simulink model "completo"  (R2022b)
settings: Solver=ode5  StartTime=0.0  StopTime=20  FixedStep=0.0001  RelTol=1e-3
InitFcn:
  | params_completo
values from neighbouring files (symbols this model uses):
  a = 1/tau    (= 1000)    [params_completo.m]
  A = [0, -a ... (first row only)    [params_completo.m]
  A_h = 0.4297    [params_completo.m]
  alpha = 40    [params_completo.m]
  b = dp/tau    (= 10000)    [params_completo.m]
  C = [1, 0]    [params_completo.m]
  k1 = 700    [params_completo.m]
  k2 = 500    [params_completo.m]
  kap1 = 1800    [params_completo.m]
  kappa = 200    [params_completo.m]
  Q = [6000 0 ... (first row only)    [params_completo.m]
  theta = 2000    [params_completo.m]
undefined symbols (not defined in the file or in its folder): B_h, cp, freq, G_h
settings Model: Creator=gerar  LastModifiedBy=Gerardo
settings SolverCC: AlgebraicLoopSolver=TrustRegion
settings DebuggingCC: UnconnectedInputMsg=warning  UnconnectedOutputMsg=warning  UnconnectedLineMsg=warning  SFMachineParentedDataDiag=warning
settings ModelReferenceCC: EnableRefExpFcnMdlSchedulingChecks=on
settings SFSimCC: CustomCodeUndefinedFunction=UseInterfaceOnly

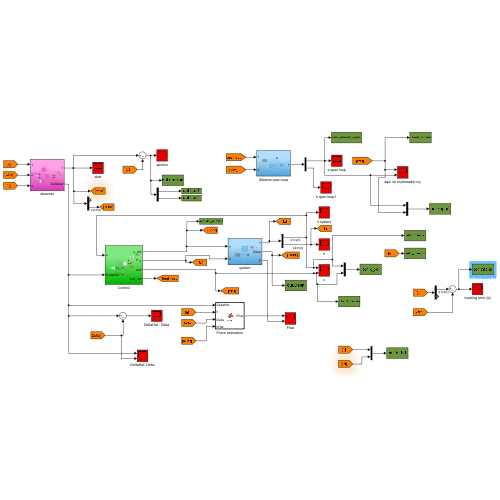
[thumbnail: Simulink's stored preview of the top-level diagram]
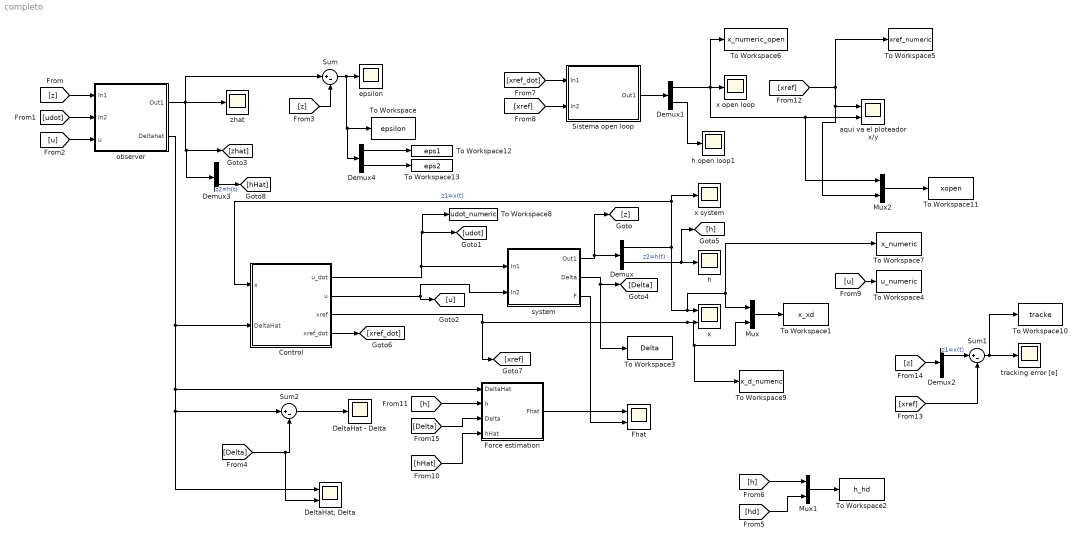
== system completo ==
  Control : Subsystem
  DeltaHat - Delta : Scope
  "DeltaHat, Delta" : Scope  NumInputPorts=2
  Demux{,1..4} (5 alike) : Demux  Outputs=2
  Fhat : Scope  NumInputPorts=2
  Force estimation : MATLAB Function  TreatAsAtomicUnit=on
  Mux : Mux  Inputs=2
  Mux1 : Mux  Inputs=2
  Mux2 : Mux  Inputs=2
  Sistema open loop : Subsystem
  Sum : Sum  Inputs=|+-
  Sum1 : Sum  Inputs=|+-
  Sum2 : Sum  Inputs=|+-
  To Workspace : ToWorkspace  VariableName=epsilon  SaveFormat=Timeseries  SampleTime=-1
  To Workspace1 : ToWorkspace  VariableName=x_xd  SaveFormat=Timeseries  SampleTime=-1
  To Workspace10 : ToWorkspace  VariableName=tracke  SaveFormat=Timeseries  SampleTime=-1
  To Workspace11 : ToWorkspace  VariableName=xopen  SaveFormat=Timeseries  SampleTime=-1
  To Workspace12 : ToWorkspace  VariableName=eps1  SaveFormat=Timeseries  SampleTime=-1
  To Workspace13 : ToWorkspace  VariableName=eps2  SaveFormat=Timeseries  SampleTime=-1
  To Workspace2 : ToWorkspace  VariableName=h_hd  SaveFormat=Timeseries  SampleTime=-1
  To Workspace3 : ToWorkspace  VariableName=Delta  SaveFormat=Timeseries  SampleTime=-1
  To Workspace4 : ToWorkspace  VariableName=u_numeric  SaveFormat=Structure  SampleTime=-1
  To Workspace5 : ToWorkspace  VariableName=xref_numeric  SaveFormat=Structure  SampleTime=-1
  To Workspace6 : ToWorkspace  VariableName=x_numeric_open  SaveFormat=Structure  SampleTime=-1
  To Workspace7 : ToWorkspace  VariableName=x_numeric  SaveFormat=Structure  SampleTime=-1
  To Workspace8 : ToWorkspace  VariableName=udot_numeric  SaveFormat=Structure  SampleTime=-1
  To Workspace9 : ToWorkspace  VariableName=x_d_numeric  SaveFormat=Structure  SampleTime=-1
  aqui va el ploteador x/y : Scope  NumInputPorts=2
  epsilon : Scope
  h : Scope
  h open loop1 : Scope
  observer : Subsystem
  system : Subsystem
  tracking error [e] : Scope
  x : Scope  NumInputPorts=2
  x open loop : Scope
  x system : Scope
  zhat : Scope
  wires:
  Control/1(u_dot) -> To Workspace8/1, [udot], system/1(In1)
  Control/2(u) -> system/2(In2), [u]
  Control/3(xref) -> [xref], To Workspace9/1, Mux/2, x/2
  Demux/2 -> [h], h/1  "z2=h(t)"
  Demux/1 -> Mux/1, To Workspace7/1, x/1, x system/1, Control/1(x)  "z1=x(t)"
  system/1(Out1) -> Demux/1, [z]
  [z] -> observer/1(In1)
  observer/1(Out1) -> Demux3/1, [zhat], zhat/1, Sum/1
  [udot] -> observer/2(In2)
  [u] -> observer/3(u)
  [z] -> Sum/2
  Sum/1 -> Demux4/1, To Workspace/1, epsilon/1
  Mux/1 -> To Workspace1/1
  [h] -> Mux1/1
  [hd] -> Mux1/2
  Mux1/1 -> To Workspace2/1
  Control/4(xref_dot) -> [xref_dot]
  [xref_dot] -> Sistema open loop/1(In1)
  [xref] -> Sistema open loop/2(In2)
  Sistema open loop/1(Out1) -> Demux1/1
  Demux1/2 -> h open loop1/1
  Demux1/1 -> To Workspace6/1, x open loop/1, Mux2/1, aqui va el ploteador x/y/2
  [u] -> To Workspace4/1
  [xref] -> To Workspace5/1, Mux2/2, aqui va el ploteador x/y/1
  Mux2/1 -> To Workspace11/1
  [z] -> Demux2/1
  Demux2/1 -> Sum1/1  "z1=x(t)"
  [xref] -> Sum1/2
  Sum1/1 -> To Workspace10/1, tracking error [e]/1
  observer/2(Deltahat) -> "DeltaHat, Delta"/1, Sum2/1, Force estimation/1(DeltaHat), Control/2(DeltaHat)
  system/2(Delta) -> To Workspace3/1, [Delta]
  [Delta] -> "DeltaHat, Delta"/2, Sum2/2
  Sum2/1 -> DeltaHat - Delta/1
  Force estimation/1(Fhat) -> Fhat/1
  Demux3/2 -> [hHat]  "z2=h(t)"
  [hHat] -> Force estimation/4(hHat)
  system/3(F) -> Fhat/2
  [h] -> Force estimation/2(h)
  [Delta] -> Force estimation/3(Delta)
  Demux4/1 -> To Workspace12/1
  Demux4/2 -> To Workspace13/1

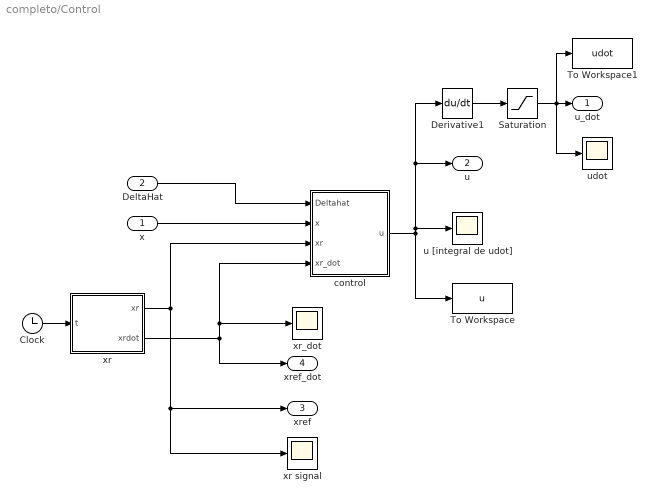
== system completo/Control ==
  x : Inport
  DeltaHat : Inport  Port=2
  Clock : Clock
  Derivative1 : Derivative
  Saturation : Saturate  UpperLimit=100  LowerLimit=-100
  To Workspace : ToWorkspace  VariableName=u  SaveFormat=Timeseries  SampleTime=-1
  To Workspace1 : ToWorkspace  VariableName=udot  SaveFormat=Timeseries  SampleTime=-1
  control : MATLAB Function  TreatAsAtomicUnit=on
  u [integral de udot] : Scope
  udot : Scope
  xr : MATLAB Function  TreatAsAtomicUnit=on
  xr signal : Scope
  xr_dot : Scope
  u_dot : Outport  VectorParamsAs1DForOutWhenUnconnected=off
  u : Outport  Port=2  VectorParamsAs1DForOutWhenUnconnected=off
  xref : Outport  Port=3  VectorParamsAs1DForOutWhenUnconnected=off
  xref_dot : Outport  Port=4  VectorParamsAs1DForOutWhenUnconnected=off
  wires:
  x/1 -> control/2(x)
  Clock/1 -> xr/1(t)
  xr/1(xr) -> xr signal/1, xref/1, control/3(xr)
  xr/2(xrdot) -> xref_dot/1, xr_dot/1, control/4(xr_dot)
  control/1(u) -> Derivative1/1, u/1, u [integral de udot]/1, To Workspace/1
  Derivative1/1 -> Saturation/1
  Saturation/1 -> To Workspace1/1, udot/1, u_dot/1
  DeltaHat/1 -> control/1(Deltahat)

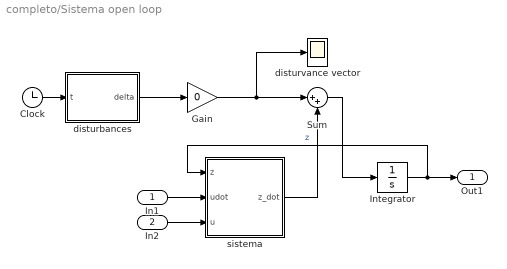
== system completo/Sistema open loop ==
  In1 : Inport
  In2 : Inport  Port=2
  Clock : Clock
  Gain : Gain  Gain=0
  Integrator : Integrator  InitialCondition=[3;-2]
  Sum : Sum  Inputs=|++
  disturbances : MATLAB Function  TreatAsAtomicUnit=on
  disturvance vector : Scope
  sistema : MATLAB Function  TreatAsAtomicUnit=on
  Out1 : Outport  VectorParamsAs1DForOutWhenUnconnected=off
  wires:
  Integrator/1 -> Out1/1, sistema/1(z)  "z"
  In1/1 -> sistema/2(udot)
  In2/1 -> sistema/3(u)
  Clock/1 -> disturbances/1(t)
  sistema/1(z_dot) -> Sum/2
  disturbances/1(delta) -> Gain/1
  Sum/1 -> Integrator/1
  Gain/1 -> Sum/1, disturvance vector/1

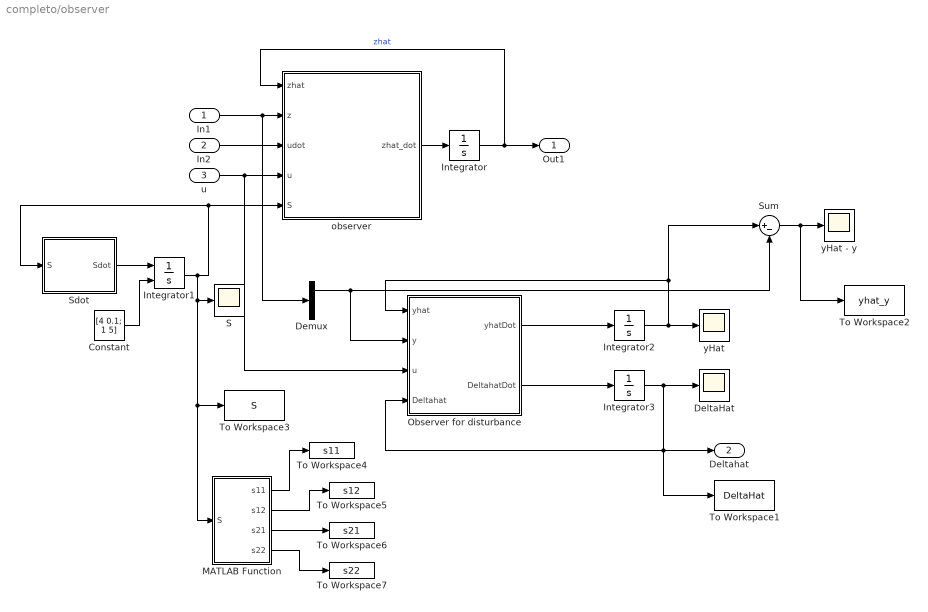
== system completo/observer ==
  In1 : Inport
  In2 : Inport  Port=2
  u : Inport  Port=3
  Constant : Constant  Value=[4 0.1; 1 5]
  DeltaHat : Scope
  Demux : Demux  Outputs=2
  Integrator : Integrator  InitialCondition=[0;0]
  Integrator1 : Integrator  InitialConditionSource=external
  Integrator2 : Integrator
  Integrator3 : Integrator
  MATLAB Function : MATLAB Function  TreatAsAtomicUnit=on
  Observer for disturbance : MATLAB Function  TreatAsAtomicUnit=on
  S : Scope
  Sdot : MATLAB Function  TreatAsAtomicUnit=on
  Sum : Sum  Inputs=|+-
  To Workspace1 : ToWorkspace  VariableName=DeltaHat  SaveFormat=Timeseries  SampleTime=-1
  To Workspace2 : ToWorkspace  VariableName=yhat_y  SaveFormat=Timeseries  SampleTime=-1
  To Workspace3 : ToWorkspace  VariableName=S  SaveFormat=Timeseries  SampleTime=-1
  To Workspace4 : ToWorkspace  VariableName=s11  SaveFormat=Timeseries  SampleTime=-1
  To Workspace5 : ToWorkspace  VariableName=s12  SaveFormat=Timeseries  SampleTime=-1
  To Workspace6 : ToWorkspace  VariableName=s21  SaveFormat=Timeseries  SampleTime=-1
  To Workspace7 : ToWorkspace  VariableName=s22  SaveFormat=Timeseries  SampleTime=-1
  observer : MATLAB Function  TreatAsAtomicUnit=on
  yHat : Scope
  yHat - y : Scope
  Out1 : Outport  VectorParamsAs1DForOutWhenUnconnected=off
  Deltahat : Outport  Port=2  VectorParamsAs1DForOutWhenUnconnected=off
  wires:
  observer/1(zhat_dot) -> Integrator/1
  Integrator/1 -> observer/1(zhat), Out1/1  "zhat"
  In1/1 -> Demux/1, observer/2(z)
  In2/1 -> observer/3(udot)
  u/1 -> Observer for disturbance/3(u), observer/4(u)
  Constant/1 -> Integrator1/2
  Sdot/1(Sdot) -> Integrator1/1
  Integrator1/1 -> MATLAB Function/1(S), To Workspace3/1, S/1, Sdot/1(S), observer/5(S)
  Observer for disturbance/1(yhatDot) -> Integrator2/1
  Observer for disturbance/2(DeltahatDot) -> Integrator3/1
  Integrator2/1 -> yHat/1, Sum/1, Observer for disturbance/1(yhat)
  Integrator3/1 -> DeltaHat/1, To Workspace1/1, Observer for disturbance/4(Deltahat), Deltahat/1
  Demux/1 -> Sum/2, Observer for disturbance/2(y)
  Sum/1 -> To Workspace2/1, yHat - y/1
  MATLAB Function/1(s11) -> To Workspace4/1
  MATLAB Function/2(s12) -> To Workspace5/1
  MATLAB Function/3(s21) -> To Workspace6/1
  MATLAB Function/4(s22) -> To Workspace7/1

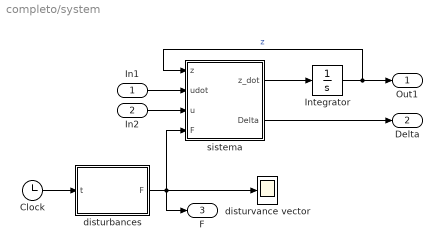
== system completo/system ==
  In1 : Inport
  In2 : Inport  Port=2
  Clock : Clock
  Integrator : Integrator  InitialCondition=[3;-2]
  disturbances : MATLAB Function  TreatAsAtomicUnit=on
  disturvance vector : Scope
  sistema : MATLAB Function  TreatAsAtomicUnit=on
  Out1 : Outport  VectorParamsAs1DForOutWhenUnconnected=off
  Delta : Outport  Port=2  VectorParamsAs1DForOutWhenUnconnected=off
  F : Outport  Port=3  VectorParamsAs1DForOutWhenUnconnected=off
  wires:
  Integrator/1 -> Out1/1, sistema/1(z)  "z"
  In1/1 -> sistema/2(udot)
  In2/1 -> sistema/3(u)
  Clock/1 -> disturbances/1(t)
  disturbances/1(F) -> F/1, sistema/4(F), disturvance vector/1
  sistema/1(z_dot) -> Integrator/1
  sistema/2(Delta) -> Delta/1

== matlab function completo/Sistema open loop/disturbances ==
  data: t input; delta output
function delta = dist(t)

delta_x = 30;
delta_h = 25*sin(t); %2*sin(t); -- causa error en el observer

delta = [delta_x ; delta_h];

== matlab function completo/Sistema open loop/sistema ==
  data: z input; udot input; u input; z_dot output; A parameter; A_h parameter; B_h parameter; G_h parameter; a parameter; b parameter
function z_dot = sys(z, udot, u, A, A_h, B_h, G_h, a, b)

gx = [ - a*z(1,1) + b*u ; 
       A_h*udot - B_h*abs(udot)*z(2,1) - G_h*udot*abs(z(2,1))];

z_dot = A*z + gx ;

== matlab function completo/observer/Sdot ==
  data: S input; Sdot output; a parameter; C parameter; theta parameter; Q parameter
function Sdot = fcn(S, a, C, theta, Q)

A_ = [ 0 -a ; 
       0  0 ];

Sdot = - theta*S - A_'*S - S*A_ + Q*(C'*C);

== matlab function completo/observer/Observer for disturbance ==
  data: yhat input; y input; u input; Deltahat input; yhatDot output; DeltahatDot output; b parameter; k1 parameter; k2 parameter; a parameter
function [yhatDot, DeltahatDot] = fcn(yhat, y, u, Deltahat, b, k1, k2, a)

yhatDot = - a*yhat + b*u + Deltahat - k1*(yhat - y);
DeltahatDot = - (yhat - y) + (k2)*(k2 - a - k1)*(yhat - y) ;

== matlab function completo/observer/MATLAB Function ==
  data: S input; s11 output; s12 output; s21 output; s22 output
function [s11, s12, s21, s22] = fcn(S)

s11 = S(1,1);
s12 = S(1,2);
s21 = S(2,1);
s22 = S(2,2);

== matlab function completo/Force estimation ==
  data: DeltaHat input; h input; Delta input; Fhat output; hHat input; cp parameter; a parameter
function Fhat = fcn(DeltaHat, h, Delta, hHat, cp, a)

Fhat = - (1/cp) * (DeltaHat/a + hHat);

== matlab function completo/system/disturbances ==
  data: t input; F output
function F = dist(t)

F = 3*sin(0.5*t);

== matlab function completo/observer/observer ==
  data: zhat input; z input; udot input; u input; S input; zhat_dot output; A parameter; A_h parameter; B_h parameter; G_h parameter; a parameter; b parameter; C parameter; Q parameter; kappa parameter
function zhat_dot = obs(zhat, z, udot, u, S, A, A_h, B_h, G_h, a, b, C, Q, kappa)

phix = [ - a*zhat(1,1) + b*u ; 
        A_h*udot - B_h*abs(udot)*zhat(2,1) - G_h*udot*abs(zhat(2,1))];

A_ = [ 0 -a ; 
       0  0 ];

zhat_dot = A_*zhat + phix - kappa* S\Q*C'*(zhat(1,1) - z(1,1));

== matlab function completo/Control/control ==
  data: Deltahat input; x input; xr input; xr_dot input; u output; kap1 parameter; a parameter; b parameter
function u = fcn(Deltahat, x, xr, xr_dot, kap1, a, b)

ex = x - xr;
%hd = (1/b) * ( - a*(ex) - kap1*sign(ex)*sqrt(abs(ex)) + a*(xr) - xr_dot + b*k*u )   ; 
u = (1/b) * ( a*x - Deltahat + xr_dot - kap1*ex );  %--- por que el termino  sign(k)????

== matlab function completo/Control/xr ==
  data: t input; xr output; alpha parameter; xrdot output; freq parameter
function [xr, xrdot] = fcn(t, alpha, freq)

xr = alpha*sin(freq*t);
xrdot = alpha*freq*cos(freq*t);

%xr = alpha;
%xrdot = 0;

== matlab function completo/system/sistema ==
  data: z input; udot input; u input; F input; z_dot output; A parameter; A_h parameter; B_h parameter; G_h parameter; a parameter; b parameter; Delta output; cp parameter
function [z_dot, Delta] = sys(z, udot, u, F, A, A_h, B_h, G_h, a, b, cp)

z_dot = [ - a*z(1,1) + b*u - a*z(2,1) - a*cp*F   ; 
         A_h*udot - B_h*abs(udot)*z(2,1) - G_h*udot*abs(z(2,1))];

% z(1,1) = x
% z(2,1) = h

Delta = - a*z(2,1) - a*cp*F ;
